simulink model "degree"  (R2020a)
settings: Solver=FixedStepDiscrete  StartTime=0.0  StopTime=360  RelTol=1e-3
PreLoadFcn:
  | A = [1:360]';
  | B = A + 120;
  | C = A + 240;
  | t=[1:360]';
settings Model: Creator=hussein  LastModifiedBy=hussein

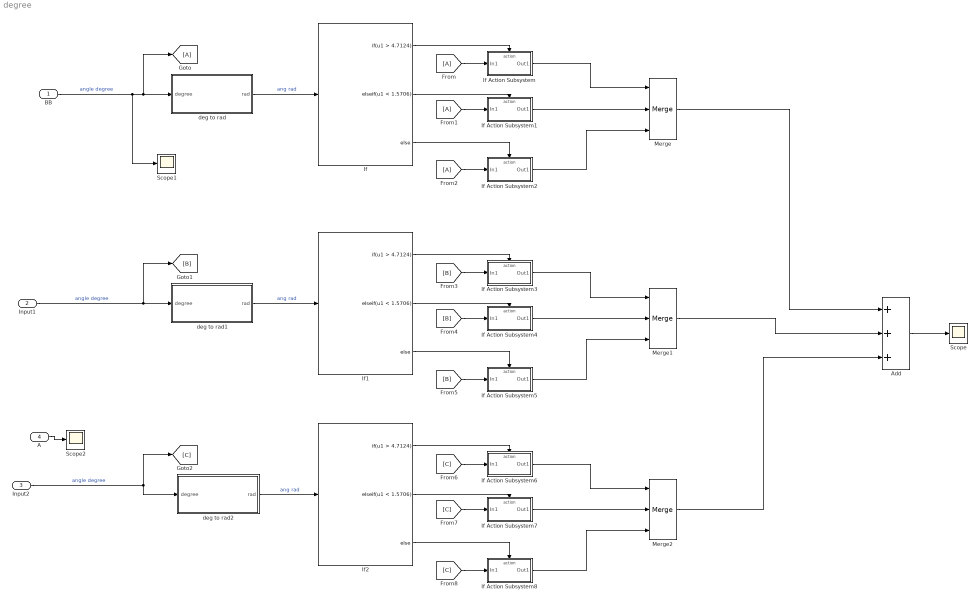
== system degree ==
  BB : Inport
  Input1 : Inport  Port=2
  Input2 : Inport  Port=3
  A : Inport  Port=4
  Add : Sum  Inputs=+++
  If : If  IfExpression=u1 > 4.7124  ElseIfExpressions=u1 < 1.5706
  If Action Subsystem : Subsystem  TreatAsAtomicUnit=on
  If Action Subsystem1 : Subsystem  TreatAsAtomicUnit=on
  If Action Subsystem2 : Subsystem  TreatAsAtomicUnit=on
  If Action Subsystem3 : Subsystem  TreatAsAtomicUnit=on
  If Action Subsystem4 : Subsystem  TreatAsAtomicUnit=on
  If Action Subsystem5 : Subsystem  TreatAsAtomicUnit=on
  If Action Subsystem6 : Subsystem  TreatAsAtomicUnit=on
  If Action Subsystem7 : Subsystem  TreatAsAtomicUnit=on
  If Action Subsystem8 : Subsystem  TreatAsAtomicUnit=on
  If1 : If  IfExpression=u1 > 4.7124  ElseIfExpressions=u1 < 1.5706
  If2 : If  IfExpression=u1 > 4.7124  ElseIfExpressions=u1 < 1.5706
  Merge : Merge  Inputs=3
  Merge1 : Merge  Inputs=3
  Merge2 : Merge  Inputs=3
  Scope : Scope
  Scope1 : Scope
  Scope2 : Scope
  deg to rad : Subsystem
  deg to rad1 : Subsystem
  deg to rad2 : Subsystem
  wires:
  If/1 -> If Action Subsystem/Action
  If/2 -> If Action Subsystem1/Action
  If/3 -> If Action Subsystem2/Action
  BB/1 -> Scope1/1, [A], deg to rad/1(degree)  "angle degree"
  deg to rad/1(rad) -> If/1  "ang rad"
  [A] -> If Action Subsystem2/1(In1)
  [A] -> If Action Subsystem1/1(In1)
  If Action Subsystem1/1(Out1) -> Merge/2
  If Action Subsystem2/1(Out1) -> Merge/3
  [A] -> If Action Subsystem/1(In1)
  If Action Subsystem/1(Out1) -> Merge/1
  If Action Subsystem3/1(Out1) -> Merge1/1
  [B] -> If Action Subsystem3/1(In1)
  [B] -> If Action Subsystem5/1(In1)
  If Action Subsystem5/1(Out1) -> Merge1/3
  If Action Subsystem4/1(Out1) -> Merge1/2
  deg to rad1/1(rad) -> If1/1  "ang rad"
  If1/1 -> If Action Subsystem3/Action
  [B] -> If Action Subsystem4/1(In1)
  If1/3 -> If Action Subsystem5/Action
  Input1/1 -> [B], deg to rad1/1(degree)  "angle degree"
  If1/2 -> If Action Subsystem4/Action
  If Action Subsystem6/1(Out1) -> Merge2/1
  [C] -> If Action Subsystem6/1(In1)
  [C] -> If Action Subsystem8/1(In1)
  If Action Subsystem8/1(Out1) -> Merge2/3
  If Action Subsystem7/1(Out1) -> Merge2/2
  deg to rad2/1(rad) -> If2/1  "ang rad"
  If2/1 -> If Action Subsystem6/Action
  [C] -> If Action Subsystem7/1(In1)
  If2/3 -> If Action Subsystem8/Action
  Input2/1 -> deg to rad2/1(degree), [C]  "angle degree"
  If2/2 -> If Action Subsystem7/Action
  Merge1/1 -> Add/2
  Merge/1 -> Add/1
  Merge2/1 -> Add/3
  Add/1 -> Scope/1
  A/1 -> Scope2/1

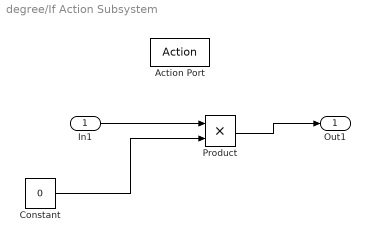
== system degree/If Action Subsystem ==
  In1 : Inport
  Action Port : ActionPort  ActionPortLabel=if(u1 > 4.7124)
  Constant : Constant  Value=0
  Product : Product
  Out1 : Outport
  wires:
  In1/1 -> Product/1
  Constant/1 -> Product/2
  Product/1 -> Out1/1

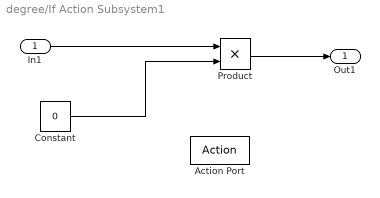
== system degree/If Action Subsystem1 ==
  In1 : Inport
  Action Port : ActionPort  ActionPortLabel=elseif(u1 < 1.5706)
  Constant : Constant  Value=0
  Product : Product
  Out1 : Outport
  wires:
  In1/1 -> Product/1
  Constant/1 -> Product/2
  Product/1 -> Out1/1

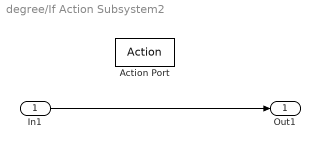
== system degree/If Action Subsystem2 ==
  In1 : Inport
  Action Port : ActionPort  ActionPortLabel=else
  Out1 : Outport
  wires:
  In1/1 -> Out1/1

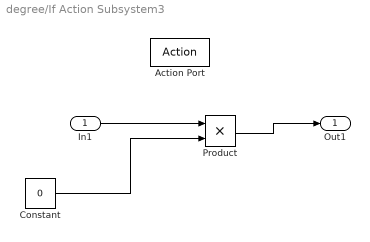
== system degree/If Action Subsystem3 ==
  In1 : Inport
  Action Port : ActionPort  ActionPortLabel=if(u1 > 4.7124)
  Constant : Constant  Value=0
  Product : Product
  Out1 : Outport
  wires:
  In1/1 -> Product/1
  Constant/1 -> Product/2
  Product/1 -> Out1/1

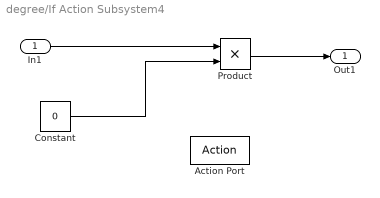
== system degree/If Action Subsystem4 ==
  In1 : Inport
  Action Port : ActionPort  ActionPortLabel=elseif(u1 < 1.5706)
  Constant : Constant  Value=0
  Product : Product
  Out1 : Outport
  wires:
  In1/1 -> Product/1
  Constant/1 -> Product/2
  Product/1 -> Out1/1

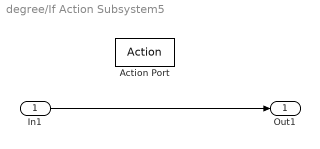
== system degree/If Action Subsystem5 ==
  In1 : Inport
  Action Port : ActionPort  ActionPortLabel=else
  Out1 : Outport
  wires:
  In1/1 -> Out1/1

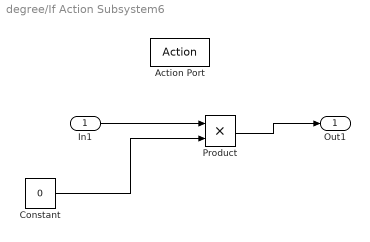
== system degree/If Action Subsystem6 ==
  In1 : Inport
  Action Port : ActionPort  ActionPortLabel=if(u1 > 4.7124)
  Constant : Constant  Value=0
  Product : Product
  Out1 : Outport
  wires:
  In1/1 -> Product/1
  Constant/1 -> Product/2
  Product/1 -> Out1/1

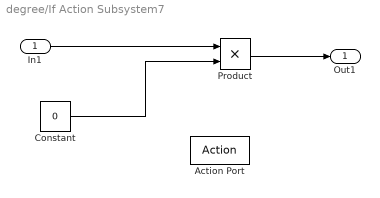
== system degree/If Action Subsystem7 ==
  In1 : Inport
  Action Port : ActionPort  ActionPortLabel=elseif(u1 < 1.5706)
  Constant : Constant  Value=0
  Product : Product
  Out1 : Outport
  wires:
  In1/1 -> Product/1
  Constant/1 -> Product/2
  Product/1 -> Out1/1

== system degree/If Action Subsystem8 ==
  In1 : Inport
  Action Port : ActionPort  ActionPortLabel=else
  Out1 : Outport
  wires:
  In1/1 -> Out1/1

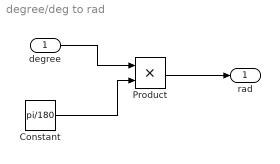
== system degree/deg to rad ==
  degree : Inport
  Constant : Constant  Value=pi/180
  Product : Product
  rad : Outport
  wires:
  degree/1 -> Product/1
  Constant/1 -> Product/2
  Product/1 -> rad/1

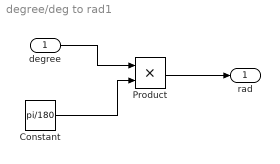
== system degree/deg to rad1 ==
  degree : Inport
  Constant : Constant  Value=pi/180
  Product : Product
  rad : Outport
  wires:
  degree/1 -> Product/1
  Constant/1 -> Product/2
  Product/1 -> rad/1

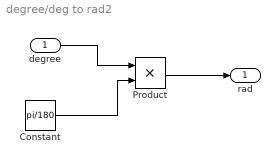
== system degree/deg to rad2 ==
  degree : Inport
  Constant : Constant  Value=pi/180
  Product : Product
  rad : Outport
  wires:
  degree/1 -> Product/1
  Constant/1 -> Product/2
  Product/1 -> rad/1
